simulink model "fuzzySimulink"  (R2025b)
settings: Solver=FixedStepAuto  StartTime=0.0  StopTime=3600  FixedStep=1  RelTol=1e-3
libraries: simulink_extras x2, fuzblock x1
settings Model: Creator=Mi-Store  LastModifiedBy=Mi-Store

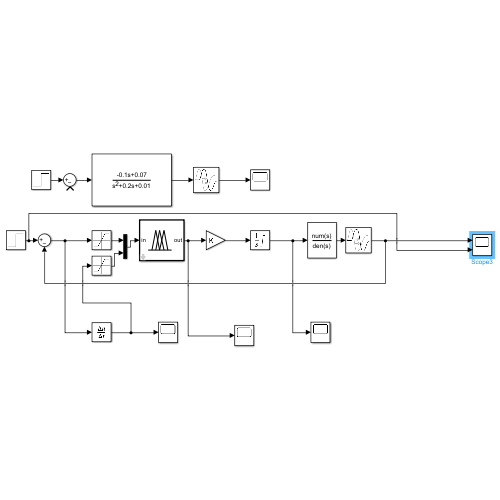
[thumbnail: Simulink's stored preview of the top-level diagram]
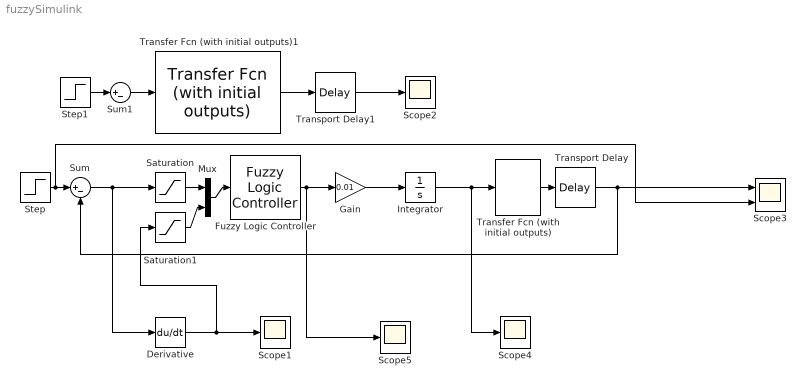
== system fuzzySimulink ==
  Derivative : Derivative
  Fuzzy Logic Controller : fuzblock/Fuzzy Logic  Controller  FIS=mamdanitype1  OutputSampleNumber=101  DataType=double  UseLookupTable=off  NumBreakpoints=10  FuzzifiedInputs=off  RuleFiringStrengths=off  RuleOutputs=off  AggregatedOutputs=off  SimulateUsing=Interpreted execution  OutOfRangeInputValueMessage=warning  NoRuleFiredMessage=warning  EmptyOutputFuzzySetMessage=warning
  Gain : Gain  Gain=0.01
  Integrator : Integrator  LimitOutput=on  UpperSaturationLimit=1  LowerSaturationLimit=-1
  Mux : Mux  Inputs=2
  Saturation : Saturate  UpperLimit=15  LowerLimit=-15
  Saturation1 : Saturate
  Scope{1..2,4..5} (4 alike) : Scope
      Scope1 settings: ActiveDisplayYMinimum=-0.027832061941056363  ActiveDisplayYMaximum=0.037952509082198577
      Scope2 settings: ActiveDisplayYMinimum=-1  ActiveDisplayYMaximum=1  DataLoggingVariableName=ScopeData2
      Scope4 settings: ActiveDisplayYMinimum=-1  ActiveDisplayYMaximum=1
      Scope5 settings: ActiveDisplayYMinimum=-1.2566162073836158  ActiveDisplayYMaximum=1.4526885876334332  DataLoggingVariableName=ScopeData4
  Scope3 : Scope  NumInputPorts=2
      settings: ActiveDisplayYMinimum=1.6920976548785431  ActiveDisplayYMaximum=2.1632235379604143  DataLoggingVariableName=ScopeData3
  Step : Step  Before=-2  After=2  SampleTime=0
  Step1 : Step  Before=-2  After=2  SampleTime=0
  Sum : Sum  Inputs=|+-
  Sum1 : Sum  Inputs=|+-
  Transfer Fcn (with initial outputs) : simulink_extras/Additional Linear/Transfer Fcn (with initial outputs)  N="[-0.1  0.07]"  D=[1 0.2 0.01]  Y0=0  U0=0
  Transfer Fcn (with initial outputs)1 : simulink_extras/Additional Linear/Transfer Fcn (with initial outputs)  N="[-0.1  0.07]"  D=[1 0.2 0.01]  Y0=0  U0=0
  Transport Delay : TransportDelay  DelayTime=4
  Transport Delay1 : TransportDelay  DelayTime=4
  wires:
  Transfer Fcn (with initial outputs)/1 -> Transport Delay/1
  Step/1 -> Scope3/2, Sum/1
  Derivative/1 -> Saturation1/1, Scope1/1
  Transport Delay1/1 -> Scope2/1
  Transfer Fcn (with initial outputs)1/1 -> Transport Delay1/1
  Sum1/1 -> Transfer Fcn (with initial outputs)1/1
  Step1/1 -> Sum1/1
  Transport Delay/1 -> Scope3/1, Sum/2
  Sum/1 -> Saturation/1, Derivative/1
  Mux/1 -> Fuzzy Logic Controller/1
  Saturation/1 -> Mux/1
  Saturation1/1 -> Mux/2
  Fuzzy Logic Controller/1 -> Scope5/1, Gain/1
  Integrator/1 -> Transfer Fcn (with initial outputs)/1, Scope4/1
  Gain/1 -> Integrator/1
